simulink model "MPPT"  (R2016a)
settings: Solver=ode3  StartTime=0.0  StopTime=1.5  FixedStep=5e-6  RelTol=1e-3
libraries: powerlib x9, re_lib x1, powerlib_meascontrol x1, simulink x1
settings Model: Creator=Emdadul Haq  LastModifiedBy=Emdadul Haq

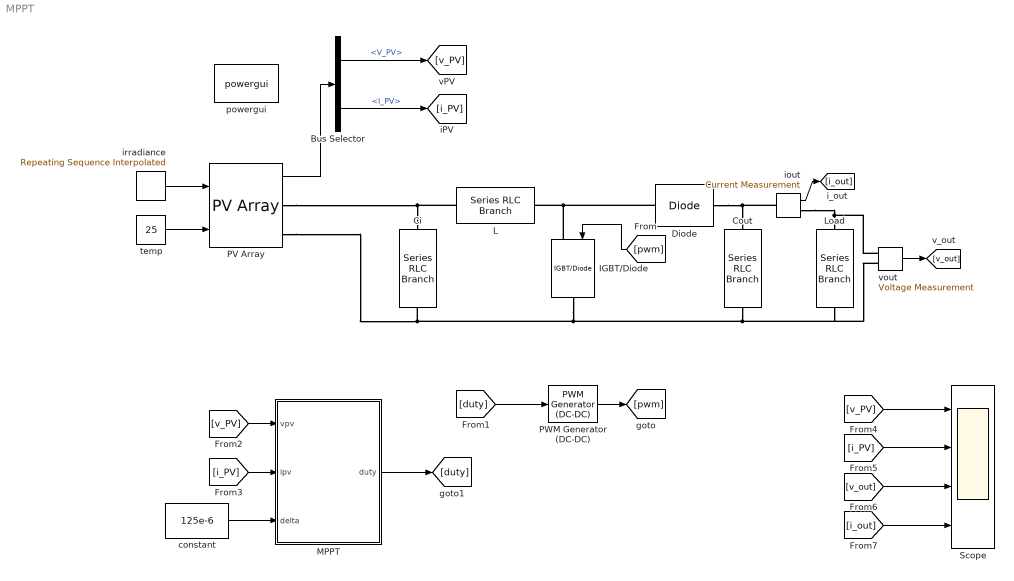
== system MPPT ==
  Bus Selector : BusSelector  OutputSignals=V_PV,I_PV
  Ci : powerlib/Elements/Series RLC Branch  LConnTagsString=__new0  RConnTagsString=__new0  BranchType=RC  Resistance=1e-4  Inductance=1e-3  SetiL0=off  InitialCurrent=0  Capacitance=100e-6  Setx0=off  InitialVoltage=0  Measurements=None
  Cout : powerlib/Elements/Series RLC Branch  LConnTagsString=__new0  RConnTagsString=__new0  BranchType=RC  Resistance=1e-4  Inductance=1e-3  SetiL0=off  InitialCurrent=0  Capacitance=100e-6  Setx0=off  InitialVoltage=0  Measurements=None
  Diode : powerlib/Power Electronics/Diode  Ron=0.001  Lon=0  Vf=0.8  IC=0  UseSnubber=off  Rs=500  Cs=250e-9  Measurements=off
  IGBT/Diode : powerlib/Power Electronics/IGBT//Diode  Ron=1e-3  Rs=1e5  Cs=inf  Measurements=off
  L : powerlib/Elements/Series RLC Branch  LConnTagsString=__new0  RConnTagsString=__new0  BranchType=RL  Resistance=.1  Inductance=2e-3  SetiL0=off  InitialCurrent=0  Capacitance=100e-6  Setx0=off  InitialVoltage=0  Measurements=None
  Load : powerlib/Elements/Series RLC Branch  LConnTagsString=__new0  RConnTagsString=__new0  BranchType=R  Resistance=20  Inductance=1e-3  SetiL0=off  InitialCurrent=0  Capacitance=100e-6  Setx0=off  InitialVoltage=0  Measurements=None
  "MPPT " : MATLAB Function  TreatAsAtomicUnit=on
  PV Array : re_lib/Solar/PV Array  Npar=2  Nser=2  PlotType=array @ 25 deg.C & specified irradiances  S_vec="[ 1000  500  100 ]"  Temp_C_vec="[ 45 25  ]"  ModuleName=1Soltech 1STH-215-P  PlotWhenSelected=off  Pm=213.15  Ncell=60  Voc=36.3  Isc=7.84  Vm=29  Im=7.35  beta_Voc_pc=-0.36099  alpha_Isc_pc=0.102  beta_Voc=-0.13104  alpha_Isc=0.007997  IL=7.8649  I0=2.9259e-10  nI=0.98117  Rsh=313.3991  Rs=0.39383  BAL=on  Tc=1e-6  Tfilter=5e-5
  PWM Generator (DC-DC) : powerlib_meascontrol/Pulse & Signal Generators/PWM Generator (DC-DC)  Fsw=5000  Ts=5e-6
  Scope : Scope  NumInputPorts=4
  constant : Constant  Value=125e-6
  iout : powerlib/Measurements/Current Measurement  PhasorSimulation=off  OutputType=Complex  PSBequivalent=0
  irradiance : simulink/Sources/Repeating Sequence Interpolated  OutValues=[0 0 300 300 500 500 1000 1000 500 500 0 0].'  TimeValues=[0 0.25 0.2501 0.5 0.501 .75 0.7501 1 1.01 1.25 1.2501 1.5].'  LookUpMeth=Interpolation-Use End Values  tsamp=0.01  OutMin=[]  OutMax=[]  OutDataTypeStr=double  OutputDataTypeScalingMode=double  OutDataType=fixdt(0,8)  OutScaling=2^-10
  powergui : powerlib/powergui  Priority=1  SimulationMode=Discrete  SolverType=Tustin/Backward Euler (TBE)  SampleTime=5e-6  frequency=60  SPID=off  DisableSnubberDevices=off  DisableRonSwitches=off  DisableVfSwitches=off  SwTol=0  DisplayEquations=off  Interpol=off  ExternalGateDelay=off  methode=off  Ts=10  FunctionMessages=off  echomessages=off  HookPort=off  EnableUseOfTLC=off  x0status=blocks  frequencyindice=0  Pbase=100e6  ErrMax=1e-4  Iterations=50  UnitsV=kV  UnitsW=MW  buscounter=0  RestoreLinks=warning  ResistiveCurrentMeasurement=off  Frange=[0:2:500]  Ylog=off  Xlog=on  ShowGrid=off  save=off  variable=ZData  structure=0  ZoomFFT=off  StartTime=0.0  cycles=1  DisplayStyle=1  fundamental=60  FreqAxis=off  MaxFrequency=1000  frequencyindicesteady=1  RmsSteady=1  display=off
  temp : Constant  Value=25
  "vout " : powerlib/Measurements/Voltage Measurement  PhasorSimulation=off  OutputType=Complex  PSBequivalent=0
  wires:
  irradiance/1 -> PV Array/1
  temp/1 -> PV Array/2
  PV Array/1 -> Bus Selector/1
  Bus Selector/1 -> [v_PV]  "<V_PV>"
  Bus Selector/2 -> [i_PV]  "<I_PV>"
  "vout "/1 -> [v_out]
  iout/1 -> [i_out]
  [pwm] -> IGBT/Diode/1
  PWM Generator (DC-DC)/1 -> [pwm]
  [duty] -> PWM Generator (DC-DC)/1
  [v_PV] -> "MPPT "/1(vpv)
  [i_PV] -> "MPPT "/2(ipv)
  constant/1 -> "MPPT "/3(delta)
  "MPPT "/1(duty) -> [duty]
  [v_PV] -> Scope/1
  [i_PV] -> Scope/2
  [v_out] -> Scope/3
  [i_out] -> Scope/4
  connections:
  PV Array/RConn1 -- L/LConn1 -- Ci/LConn1
  PV Array/RConn2 -- "vout "/LConn2 -- Load/RConn1 -- Cout/RConn1 -- IGBT/Diode/RConn1 -- Ci/RConn1
  IGBT/Diode/LConn1 -- L/RConn1 -- Diode/LConn1
  Diode/RConn1 -- Cout/LConn1 -- iout/LConn1
  iout/RConn1 -- "vout "/LConn1 -- Load/LConn1

== matlab function MPPT/MPPT  ==
  data: vpv input; duty output; ipv input; delta input
function duty = MPPT_algorithm(vpv,ipv,delta)
duty_init =0.1;
duty_min =0;
duty_max =.85;

persistent Vold Pold duty_old;

if isempty(Vold)
    Vold=0;
    Pold=0;
    duty_old=duty_init;
end
P=vpv*ipv;
dV=vpv-Vold;
dP=P-Pold;

if dP ~= 0 && vpv>30
    if dP<0
        if dV<0
            duty= duty_old - delta;
        else
            duty= duty_old + delta;
        end
    else
        if dV < 0
            duty = duty_old + delta;
        else
            duty = duty_old - delta;
        end
    end
else
    duty = duty_old;
end

if
    duty >= duty_max
    duty = duty_max;
    
elseif
    duty<duty_min
    duty = duty_min;
end

duty_old = duty;
Vold =vpv;
Pold=P;
